simulink model "Subsystem"  (R2020a)
settings: Solver=VariableStepAuto  StartTime=0.0  StopTime=10.0  RelTol=1e-3
settings Model: Creator=Riyansh  LastModifiedBy=Riyansh
settings DataIOCC: SaveOutput=off  SaveTime=off

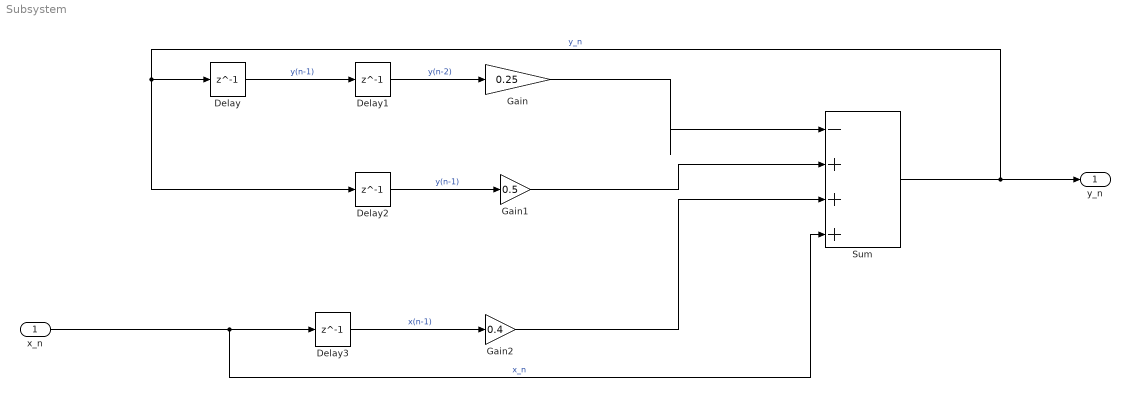
== system Subsystem ==
  x_n : Inport  OutDataTypeStr=double  PortDimensions=1  SampleTime=[0,1]
  Delay{,1..3} (4 alike) : Delay  DelayLength=1
  Gain : Gain  Gain=0.25
  Gain1 : Gain  Gain=0.5
  Gain2 : Gain  Gain=0.4
  Sum : Sum  Inputs=|-+++
  y_n : Outport  OutDataTypeStr=double  PortDimensions=1  SampleTime=[0,1]
  wires:
  Gain2/1 -> Sum/3
  Delay2/1 -> Gain1/1  "y(n-1)"
  Sum/1 -> Delay2/1, Delay/1, y_n/1  "y_n"
  Delay1/1 -> Gain/1  "y(n-2)"
  Delay3/1 -> Gain2/1  "x(n-1)"
  Gain1/1 -> Sum/2
  Gain/1 -> Sum/1
  x_n/1 -> Delay3/1, Sum/4  "x_n"
  Delay/1 -> Delay1/1  "y(n-1)"
